simulink model "mass_spring_dumper"  (R2021a)
settings: Solver=VariableStepAuto  StartTime=0.0  StopTime=10.0  MaxStep=1e-3  RelTol=1e-3
values from neighbouring files (symbols this model uses):
  b = 10    [dumber_script.m]
  k = 400    [dumber_script.m]
  m = massvalue(i)    [dumber_script.m]
  x0 = 1    [dumber_script.m]
settings Model: Creator=yasso  LastModifiedBy=yasso
settings DataIOCC: SaveFormat=StructureWithTime

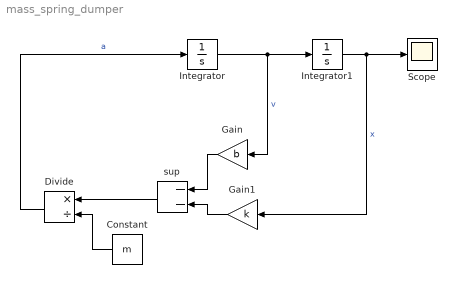
== system mass_spring_dumper ==
  Constant : Constant  Value=m
  Divide : Product  Inputs=*/
  Gain : Gain  Gain=b
  Gain1 : Gain  Gain=k
  Integrator : Integrator
  Integrator1 : Integrator  InitialCondition=x0
  Scope : Scope
  sup : Sum  Inputs=--
  wires:
  Divide/1 -> Integrator/1  "a"
  Integrator/1 -> Gain/1, Integrator1/1  "v"
  Integrator1/1 -> Gain1/1, Scope/1  "x"
  Gain/1 -> sup/1
  Gain1/1 -> sup/2
  sup/1 -> Divide/1
  Constant/1 -> Divide/2
